simulink model "modelsim"  (R2020b)
settings: Solver=VariableStepAuto  StartTime=0.0  StopTime=10.0  RelTol=1e-3
settings Model: Creator=spira  LastModifiedBy=spira

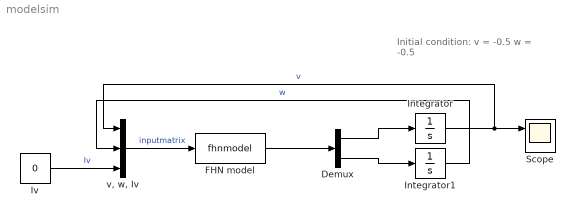
== system modelsim ==
  note: Initial condition:
      | v = -0.5
      | w = -0.5
  Demux : Demux  Outputs=2
  FHN model : MATLABFcn  MATLABFcn=fhnmodel  OutputDimensions=1
  Integrator : Integrator  InitialCondition=-0.5
  Integrator1 : Integrator  InitialCondition=-0.5
  Iv : Constant  Value=0
  Scope : Scope  NumInputPorts=2
  "v, w, Iv" : Mux  Inputs=3
  wires:
  Integrator/1 -> "v, w, Iv"/1, Scope/1  "v"
  "v, w, Iv"/1 -> FHN model/1  "inputmatrix"
  Integrator1/1 -> "v, w, Iv"/2  "w"
  Iv/1 -> "v, w, Iv"/3  "Iv"
  FHN model/1 -> Demux/1
  Demux/1 -> Integrator/1
  Demux/2 -> Integrator1/1
